simulink model "SquareWaveSumOfSineWaves_MathFunction_LowPassFilter"  (R2015b)
settings: Solver=VariableStepAuto  StartTime=0.0  StopTime=50.0  MaxStep=1.0E-3  MinStep=1.0E-4  RelTol=1e-3
libraries: dsparch4 x1
settings Model: Creator=mihai.ciobanu  LastModifiedBy=mihai.ciobanu

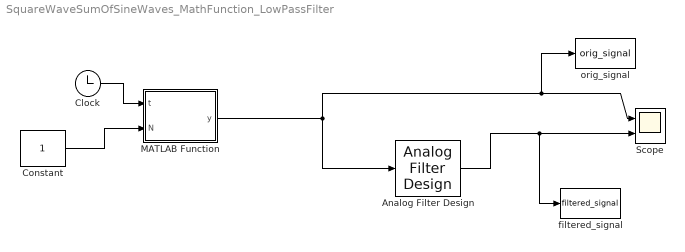
== system SquareWaveSumOfSineWaves_MathFunction_LowPassFilter ==
  Analog Filter Design : dsparch4/Analog Filter Design  method=Butterworth  filttype=Lowpass  N=1  Wlo=2*pi*10  Whi=80  Rp=2  Rs=40
  Clock : Clock
  Constant : Constant
  MATLAB Function : MATLAB Function  TreatAsAtomicUnit=on
  Scope : Scope  NumInputPorts=2
  filtered_signal : ToWorkspace  VariableName=filtered_signal  SaveFormat=Timeseries  SampleTime=1.0E-3
  orig_signal : ToWorkspace  VariableName=orig_signal  SaveFormat=Timeseries  SampleTime=1.0E-3
  wires:
  Constant/1 -> MATLAB Function/2(N)
  Clock/1 -> MATLAB Function/1(t)
  MATLAB Function/1(y) -> Analog Filter Design/1, orig_signal/1, Scope/1
  Analog Filter Design/1 -> filtered_signal/1, Scope/2

== matlab function SquareWaveSumOfSineWaves_MathFunction_LowPassFilter/MATLAB Function ==
  data: t input; N input; y output
function y = fcn(t, N)
%#codegen
y=0;
for K=1:2:N
    Frad = K/(2*pi);
    y = y+ 1/Frad*sin(Frad*t);
    %y = y+ (1/K)*sin(K*t);    
end
